simulink model "test2"  (Simulink 9.0)
settings: Solver=VariableStepAuto  StartTime=0.0  StopTime=10.0  RelTol=1e-3
settings Model: SuppressorTable=22 serialization::archive 11 0 6 0 0 0 11 0  Creator=flosch  LastModifiedBy=flosch
settings DataIOCC: SaveFormat=Dataset
settings OptimizationCC: LifeSpan=auto
settings DebuggingCC: UnderspecifiedInitializationDetection=Simplified  MergeDetectMultiDrivingBlocksExec=error  SFUnexpectedBacktrackingDiag=error  SFNoUnconditionalDefaultTransitionDiag=error  SFExecutionAtInitializationDiag=warning
settings HardwareCC: ProdBitPerPointer=64  ProdBitPerSizeT=64  ProdBitPerPtrDiffT=64  ProdLargestAtomicFloat=Float  ProdIntDivRoundTo=Zero  ProdEndianess=LittleEndian  ProdWordSize=64  ProdHWDeviceType=Intel->x86-64 (Windows64)
settings ModelReferenceCC: PropagateSignalLabelsOutOfModel=on
settings CodeAppCC: StateflowObjectComments=off
settings GRTTargetCC: TargetLangStandard=C99 (ISO)
settings ConfigComp: CovMetricSettings=dwe  CovHtmlReporting=off  CovSaveCumulativeToWorkspaceVar=off  CovSaveSingleToWorkspaceVar=off  CovExternalEMLEnable=on

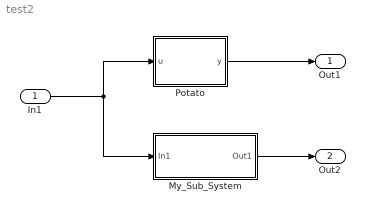
== system test2 ==
  In1 : Inport
  My_Sub_System : Subsystem
  Potato : MATLAB Function  TreatAsAtomicUnit=on
  Out1 : Outport
  Out2 : Outport  Port=2
  wires:
  In1/1 -> My_Sub_System/1(In1), Potato/1(u)
  Potato/1(y) -> Out1/1
  My_Sub_System/1(Out1) -> Out2/1

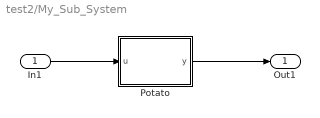
== system test2/My_Sub_System ==
  In1 : Inport
  Potato : MATLAB Function  TreatAsAtomicUnit=on
  Out1 : Outport
  wires:
  In1/1 -> Potato/1(u)
  Potato/1(y) -> Out1/1

== matlab function My_Sub_System/Potato ==
  data: u input double; y output double
function y = fcn(u)
% This is in the subsystem
y = u;

== matlab function Potato ==
  data: u input double; y output double
function y = fcn(u)
% This is in test2
y = u;
